simulink model "fu_adrc2_2018a"  (R2018a)
settings: Solver=VariableStepAuto  StartTime=0.0  StopTime=Tsim  RelTol=1e-3
values from neighbouring files (symbols this model uses):
  L = Lm    (= 0.3)    [ex2_fu.m]
  Lm = 0.3    [ex2_fu.m]
  Tpert = 10    [ex2_fu.m]
  Truido = 20    [ex2_fu.m]
  Ts = 0.05    [ex2_fu.m]
libraries: cstblocks x4, simulink x1
settings Model: Creator=rene  LastModifiedBy=Vasco
settings DebuggingCC: UnconnectedInputMsg=none  UnconnectedOutputMsg=none  UnconnectedLineMsg=none  LibraryContextMissingDiagnostic=warning
settings SFSimCC: SimUseLocalCustomCode=on
settings RTWCC: RTWUseLocalCustomCode=on

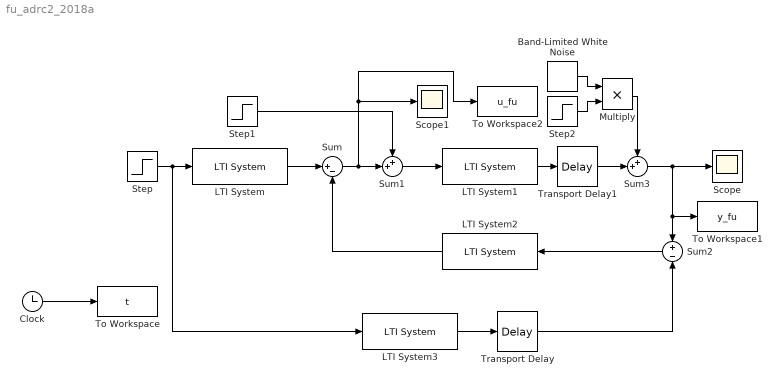
== system fu_adrc2_2018a ==
  Band-Limited White Noise : simulink/Sources/Band-Limited White Noise  Cov=1e-7  Ts=Ts  seed=[23341]
  Clock : Clock
  LTI System : cstblocks/LTI System  sys=Cr  IC=[]
  LTI System1 : cstblocks/LTI System  sys=Gp  IC=[]
  LTI System2 : cstblocks/LTI System  sys=K  IC=[]
  LTI System3 : cstblocks/LTI System  sys=N  IC=[]
  Multiply : Product
  Scope : Scope
  Scope1 : Scope
  Step : Step  Time=0  SampleTime=0
  Step1 : Step  Time=Tpert  After=-1  SampleTime=0
  Step2 : Step  Time=Truido  SampleTime=0
  Sum : Sum  Inputs=|+-
  Sum1 : Sum  Inputs=++|
  Sum2 : Sum  Inputs=+|-
  Sum3 : Sum  Inputs=++|
  To Workspace : ToWorkspace  VariableName=t  SampleTime=Ts
  To Workspace1 : ToWorkspace  VariableName=y_fu  SampleTime=Ts
  To Workspace2 : ToWorkspace  VariableName=u_fu  SampleTime=Ts
  Transport Delay : TransportDelay  DelayTime=Lm
  Transport Delay1 : TransportDelay  DelayTime=L
  wires:
  Step/1 -> LTI System3/1, LTI System/1
  LTI System/1 -> Sum/1
  Step1/1 -> Sum1/1
  Sum/1 -> Sum1/2, Scope1/1, To Workspace2/1
  Sum1/1 -> LTI System1/1
  LTI System1/1 -> Transport Delay1/1
  Sum2/1 -> LTI System2/1
  LTI System2/1 -> Sum/2
  LTI System3/1 -> Transport Delay/1
  Transport Delay/1 -> Sum2/2
  Clock/1 -> To Workspace/1
  Transport Delay1/1 -> Sum3/2
  Sum3/1 -> To Workspace1/1, Sum2/1, Scope/1
  Multiply/1 -> Sum3/1
  Step2/1 -> Multiply/2
  Band-Limited White Noise/1 -> Multiply/1
